simulink model "bruit_TD2"  (Simulink 8.6)
settings: Solver=ode45  StartTime=0.0  StopTime=t_sim  RelTol=1e-3
values from neighbouring files (symbols this model uses):
  ts = 0.000001    (= 1e-06)    [main.m]
libraries: simulink x1
settings Model: Creator=mailly  LastModifiedBy=mailly
settings OptimizationCC: ExpressionDepthLimit=128  InitFltsAndDblsToZero=on
settings DebuggingCC: SaveWithParameterizedLinksMsg=none  SignalResolutionControl=TryResolveAllWithWarning  MultiTaskDSMMsg=warning  MultiTaskCondExecSysMsg=none  FcnCallInpInsideContextMsg=UseLocalSettings  StateNameClashWarn=none  StrictBusMsg=None
settings GRTTargetCC: TargetFcnLib=ansi_tfl_tmw.mat  GeneratePreprocessorConditionals=Use local settings

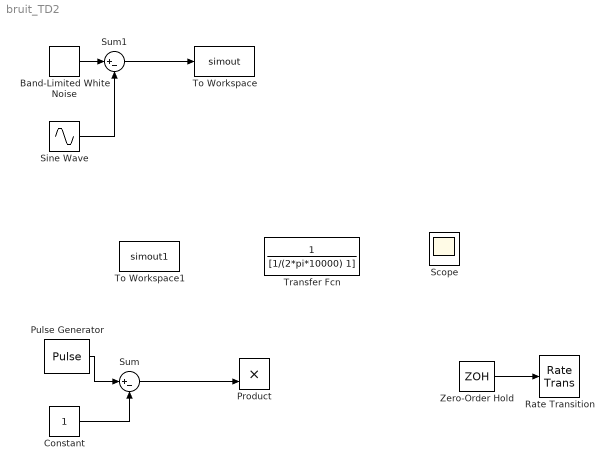
== system bruit_TD2 ==
  Band-Limited White Noise : simulink/Sources/Band-Limited White Noise  Cov=[0]  Ts=ts  seed=[23341]
  Constant : Constant
  Product : Product  SampleTime=0  RndMeth=Zero
  Pulse Generator : DiscretePulseGenerator  PulseType=Time based  Amplitude=2  Period=1/20  PulseWidth=50
  Rate Transition : RateTransition
  Scope : Scope  NumInputPorts=2
  Sine Wave : Sin  Amplitude=1e-6  Frequency=2*pi*10  SampleTime=0
  Sum : Sum  Inputs=|+-
  Sum1 : Sum  Inputs=|+-
  To Workspace : ToWorkspace  VariableName=simout  SampleTime=ts
  To Workspace1 : ToWorkspace  VariableName=simout1  SampleTime=ts
  Transfer Fcn : TransferFcn  Denominator=[1/(2*pi*10000) 1]
  Zero-Order Hold : ZeroOrderHold  SampleTime=1/200
  wires:
  Constant/1 -> Sum/2
  Pulse Generator/1 -> Sum/1
  Sum/1 -> Product/2
  Zero-Order Hold/1 -> Rate Transition/1
  Band-Limited White Noise/1 -> Sum1/1
  Sine Wave/1 -> Sum1/2
  Sum1/1 -> To Workspace/1
